simulink model "Q1_W2"  (R2020b)
settings: Solver=VariableStepAuto  StartTime=0.0  StopTime=10.0  RelTol=1e-3
settings Model: Creator=hp  LastModifiedBy=hp

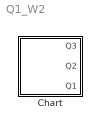
== system Q1_W2 ==
  Chart : Stateflow chart  TreatAsAtomicUnit=on

== stateflow chart Q1_W2/Chart ==
  state D_FF2
    (default) -> (junction 20) : {Q2=Q1xorQ2(Q1,Q2)}
  state D_FF1
    (default) -> (junction 25) : {Q1=Q2norQ3(Q1,Q2)}
  state D_FF3
    (default) -> (junction 12) : {Q3=Q1andQ2(Q1,Q2)}
  (default) -> D_FF3
  D_FF1 -> D_FF3 : [CLK==1]
  D_FF3 -> D_FF2 : [CLK==1]
  D_FF2 -> D_FF1 : [CLK==1]
  data: Q11 function_input; Q21 function_input; Q21 function_output; Q11 function_input; Q21 function_input; Q11 function_output; Q11 function_input; Q21 function_input; Q31 function_output; Q3 output; Q2 output; Q1 output
  function Q21=Q1xorQ2(Q11,Q21):
    | function Q21=Q1xorQ2(Q11,Q21)
    | 
    | aVarTruthTableCondition_1 = false;
    | aVarTruthTableCondition_2 = false;
    | 
    | 
    | % input from d1 flip-flop
    | 
    | aVarTruthTableCondition_1 = logical(Q11==0);
    | 
    | % input from d2 flip-flop
    | 
    | aVarTruthTableCondition_2 = logical(Q21==0);
    | 
    | if (aVarTruthTableCondition_1 && aVarTruthTableCondition_2)
    |     A1();
    | elseif (aVarTruthTableCondition_1 && ~aVarTruthTableCondition_2)
    |     A2();
    | elseif (~aVarTruthTableCondition_1 && aVarTruthTableCondition_2)
    |     A2();
    | else % Default
    |     A1();
    | end
    | 
    | function A1()
    | 
    | % output of D2 flip flop is 0
    | 
    | Q21=0;
    | 
    | function A2()
    | 
    | % output of D2 flip flip is 1
    | 
    | Q21=1;
  function Q11=Q2norQ3(Q11,Q21):
    | function Q11=Q2norQ3(Q11,Q21)
    | 
    | aVarTruthTableCondition_1 = false;
    | aVarTruthTableCondition_2 = false;
    | 
    | 
    | % input from d3 flip-flop
    | 
    | aVarTruthTableCondition_1 = logical(Q31==0);
    | 
    | % input from d2 flip-flop
    | 
    | aVarTruthTableCondition_2 = logical(Q21==0);
    | 
    | if (aVarTruthTableCondition_1 && aVarTruthTableCondition_2)
    |     A2();
    | elseif (aVarTruthTableCondition_1 && ~aVarTruthTableCondition_2)
    |     A1();
    | elseif (~aVarTruthTableCondition_1 && aVarTruthTableCondition_2)
    |     A1();
    | else % Default
    |     A1();
    | end
    | 
    | function A1()
    | 
    | % output of D3 flip flop is 0
    | 
    | Q11=0;
    | 
    | function A2()
    | 
    | % output of D3 flip flip is 1
    | 
    | Q11=1;
  function Q31=Q1andQ2(Q11,Q21):
    | function Q31=Q1andQ2(Q11,Q21)
    | 
    | aVarTruthTableCondition_1 = false;
    | aVarTruthTableCondition_2 = false;
    | 
    | 
    | % input from d1 flip-flop
    | 
    | aVarTruthTableCondition_1 = logical(Q11==0);
    | 
    | % input from d2 flip-flop
    | 
    | aVarTruthTableCondition_2 = logical(Q21==0);
    | 
    | if (aVarTruthTableCondition_1 && aVarTruthTableCondition_2)
    |     A1();
    | elseif (aVarTruthTableCondition_1 && ~aVarTruthTableCondition_2)
    |     A1();
    | elseif (~aVarTruthTableCondition_1 && aVarTruthTableCondition_2)
    |     A1();
    | else % Default
    |     A2();
    | end
    | 
    | function A1()
    | 
    | % output of D3 flip flop is 0
    | 
    | Q31=0;
    | 
    | function A2()
    | 
    | % output of D3 flip flip is 1
    | 
    | Q31=1;
